simulink subsystem "shortest_angle_diff"  (R2022b)
settings: Solver=VariableStepAuto  StartTime=0.0  StopTime=10.0  RelTol=1e-3
settings Model: Creator=papaveneti  LastModifiedBy=papaveneti

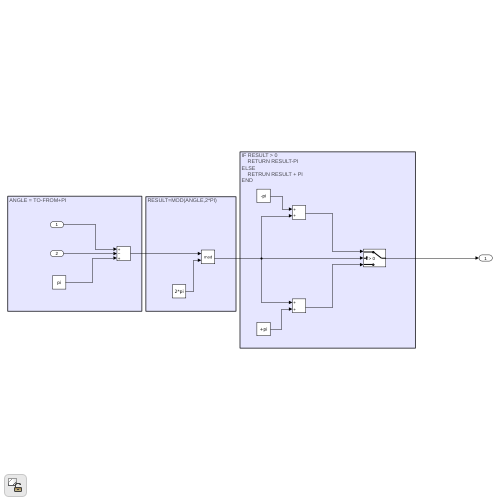
[thumbnail: Simulink's stored preview of the top-level diagram]
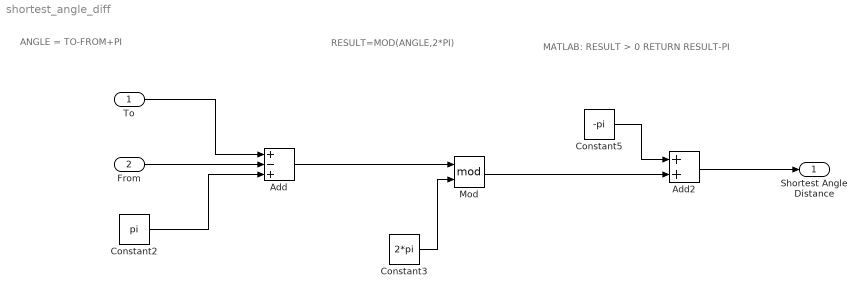
== system shortest_angle_diff ==
  note: MATLAB: RESULT > 0
      | RETURN RESULT-PI
  note: RESULT=MOD(ANGLE,2*PI)
  note: ANGLE = TO-FROM+PI
  To : Inport
  From : Inport  Port=2
  Add : Sum  Inputs=+-+
  Add2 : Sum
  Constant2 : Constant  Value=pi
  Constant3 : Constant  Value=2*pi
  Constant5 : Constant  Value=-pi
  Mod : Math  Operator=mod
  Shortest Angle Distance : Outport
  wires:
  From/1 -> Add/2
  Constant3/1 -> Mod/2
  To/1 -> Add/1
  Constant2/1 -> Add/3
  Add2/1 -> Shortest Angle Distance/1
  Constant5/1 -> Add2/1
  Mod/1 -> Add2/2
  Add/1 -> Mod/1
